simulink model "NonLinMod8"  (Simulink 8.1)
settings: Solver=ode23s  StartTime=0.0  StopTime=3  RelTol=1e-2
values from neighbouring files (symbols this model uses):
  A = [-3 1;-8 -9]    [main.m]
  a = 0.01    [main.m]
  B = [0.5; 0]    [main.m]
  b = 1    [main.m]
  g = 0.8    [main.m]
  K = [9 4]    [main.m]
  xs0 = [1.9; 0]    [main.m]
libraries: simulink x1
settings Model: Creator=paul  LastModifiedBy=paul
settings SolverCC: ConsecutiveZCsStepRelTol=100*128*eps
settings DataIOCC: SignalLoggingSaveFormat=Dataset
settings OptimizationCC: ExpressionDepthLimit=128
settings DebuggingCC: SolverPrmCheckMsg=none  FcnCallInpInsideContextMsg=EnableAllAsError
settings GRTTargetCC: CombineOutputUpdateFcns=on  GRTInterface=off

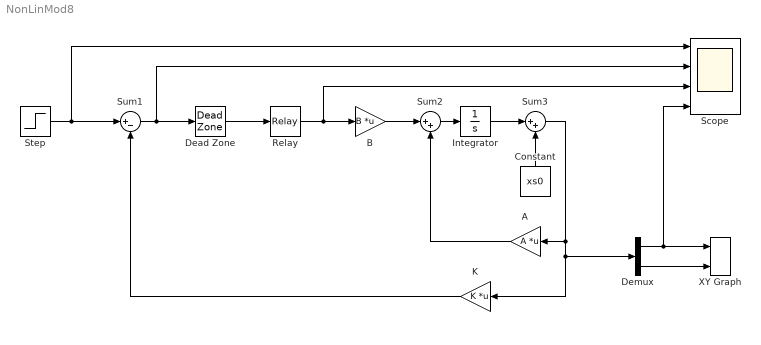
== system NonLinMod8 ==
  A : Gain  Gain=A  Multiplication=Matrix(K*u)
  B : Gain  Gain=B  Multiplication=Matrix(K*u)
  Constant : Constant  Value=xs0
  Dead Zone : DeadZone  LowerValue=-a  UpperValue=a  SaturateOnIntegerOverflow=on
  Demux : Demux  Outputs=2
  Integrator : Integrator
  K : Gain  Gain=K  Multiplication=Matrix(K*u)
  Relay : Relay  OffSwitchValue=-eps  OnOutputValue=b  OffOutputValue=-b
  Scope : Scope  NumInputPorts=4
      settings: TimeRange=2  YMin=2.85~-0.075~-1.5~-2  YMax=3.15~0.075~1.5~2  MaxDataPoints=15000
  Step : Step  Time=0.1  After=g  SampleTime=0
  Sum1 : Sum  Inputs=|+-
  Sum2 : Sum  Inputs=|++
  Sum3 : Sum  Inputs=|++
  XY Graph : simulink/Sinks/XY Graph  xmin=-1  xmax=2  ymin=-1  ymax=1.8  st=-1
  wires:
  K/1 -> Sum1/2
  Demux/2 -> XY Graph/2
  Demux/1 -> Scope/4, XY Graph/1
  B/1 -> Sum2/1
  Sum2/1 -> Integrator/1
  Integrator/1 -> Sum3/1
  A/1 -> Sum2/2
  Step/1 -> Sum1/1, Scope/1
  Sum3/1 -> Demux/1, K/1, A/1
  Constant/1 -> Sum3/2
  Relay/1 -> Scope/3, B/1
  Sum1/1 -> Dead Zone/1, Scope/2
  Dead Zone/1 -> Relay/1
